simulink model "aprendiendoUsarFuzzyLogicController"  (R2024b)
settings: Solver=VariableStepAuto  StartTime=0.0  StopTime=10.0  RelTol=1e-3
libraries: fuzblock x1, simulink x1
settings Model: Creator=user  LastModifiedBy=user

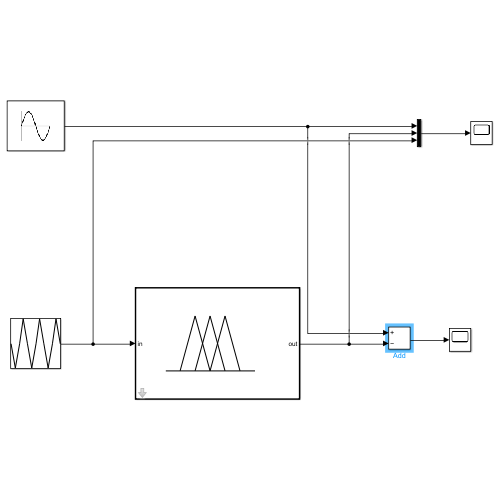
[thumbnail: Simulink's stored preview of the top-level diagram]
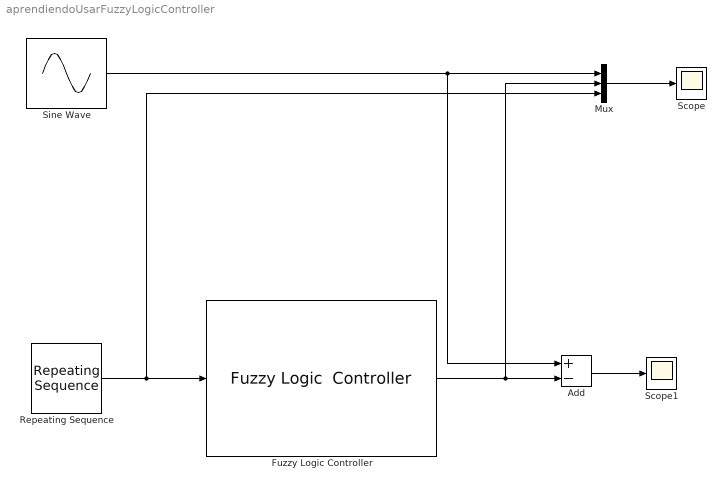
== system aprendiendoUsarFuzzyLogicController ==
  Add : Sum  Inputs=+-
  Fuzzy Logic Controller : fuzblock/Fuzzy Logic  Controller  FIS='tirangularA2seno.fis'  OutputSampleNumber=101  DataType=double  FuzzifiedInputs=off  RuleFiringStrengths=off  RuleOutputs=off  AggregatedOutputs=off  SimulateUsing=Interpreted execution  OutOfRangeInputValueMessage=warning  NoRuleFiredMessage=warning  EmptyOutputFuzzySetMessage=warning
  Mux : Mux  Inputs=3
  Repeating Sequence : simulink/Sources/Repeating Sequence  rep_seq_t=[0 2 4 6 8]  rep_seq_y=[0 -1 0 1 0]
  Scope : Scope
  Scope1 : Scope
  Sine Wave : Sin  Frequency=pi/4  Phase=pi  SampleTime=0
  wires:
  Repeating Sequence/1 -> Mux/3, Fuzzy Logic Controller/1
  Sine Wave/1 -> Add/1, Mux/1
  Add/1 -> Scope1/1
  Fuzzy Logic Controller/1 -> Mux/2, Add/2
  Mux/1 -> Scope/1
